simulink model "puma560_steadystate"  (R2015a)
settings: Solver=ode45  StartTime=0.0  StopTime=10.0  RelTol=1e-3
libraries: robotlib x8
settings Model: Creator=jwcjdenissen  LastModifiedBy=jwcjdenissen

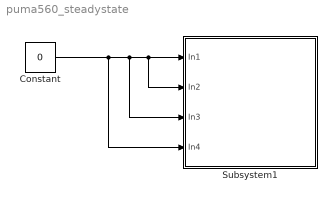
== system puma560_steadystate ==
  Constant : Constant  Value=0
  Subsystem1 : Subsystem
  wires:
  Constant/1 -> Subsystem1/1(In1), Subsystem1/2(In2), Subsystem1/3(In3), Subsystem1/4(In4)

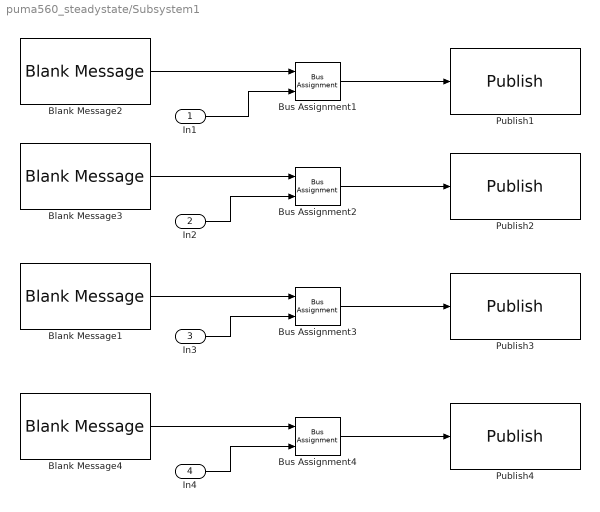
== system puma560_steadystate/Subsystem1 ==
  In1 : Inport
  In2 : Inport  Port=2
  In3 : Inport  Port=3
  In4 : Inport  Port=4
  Blank Message{1..4} (4 alike) : robotlib/Blank Message  SourceLibraryInfo=This block requires Robotics System Toolbox  messageType=std_msgs/Float64  SampleTime=inf
  Bus Assignment{1..4} (4 alike) : BusAssignment  AssignedSignals=Data
  Publish1 : robotlib/Publish  SourceLibraryInfo=This block requires Robotics System Toolbox  topicSource=Specify your own  topic=/puma560/joint_2_position_controller/command  messageType=std_msgs/Float64  messageQueueLength=1
  Publish2 : robotlib/Publish  SourceLibraryInfo=This block requires Robotics System Toolbox  topicSource=Specify your own  topic=/puma560/joint_3_position_controller/command  messageType=std_msgs/Float64  messageQueueLength=1
  Publish3 : robotlib/Publish  SourceLibraryInfo=This block requires Robotics System Toolbox  topicSource=Specify your own  topic=/puma560/joint_4_position_controller/command  messageType=std_msgs/Float64  messageQueueLength=1
  Publish4 : robotlib/Publish  SourceLibraryInfo=This block requires Robotics System Toolbox  topicSource=Specify your own  topic=/puma560/joint_5_position_controller/command  messageType=std_msgs/Float64  messageQueueLength=1
  wires:
  In1/1 -> Bus Assignment1/2
  In4/1 -> Bus Assignment4/2
  Blank Message4/1 -> Bus Assignment4/1
  Bus Assignment4/1 -> Publish4/1
  In3/1 -> Bus Assignment3/2
  Blank Message1/1 -> Bus Assignment3/1
  Bus Assignment3/1 -> Publish3/1
  In2/1 -> Bus Assignment2/2
  Blank Message3/1 -> Bus Assignment2/1
  Bus Assignment2/1 -> Publish2/1
  Blank Message2/1 -> Bus Assignment1/1
  Bus Assignment1/1 -> Publish1/1
